simulink model "SimulinkDiagram"  (R2019a)
settings: Solver=VariableStepAuto  StartTime=0.0  StopTime=10.0  RelTol=1e-3
undefined symbols (not defined in the file): DesiredPose, DesiredTwist
libraries: simulink x4
settings Model: Creator=Amador  LastModifiedBy=Amador

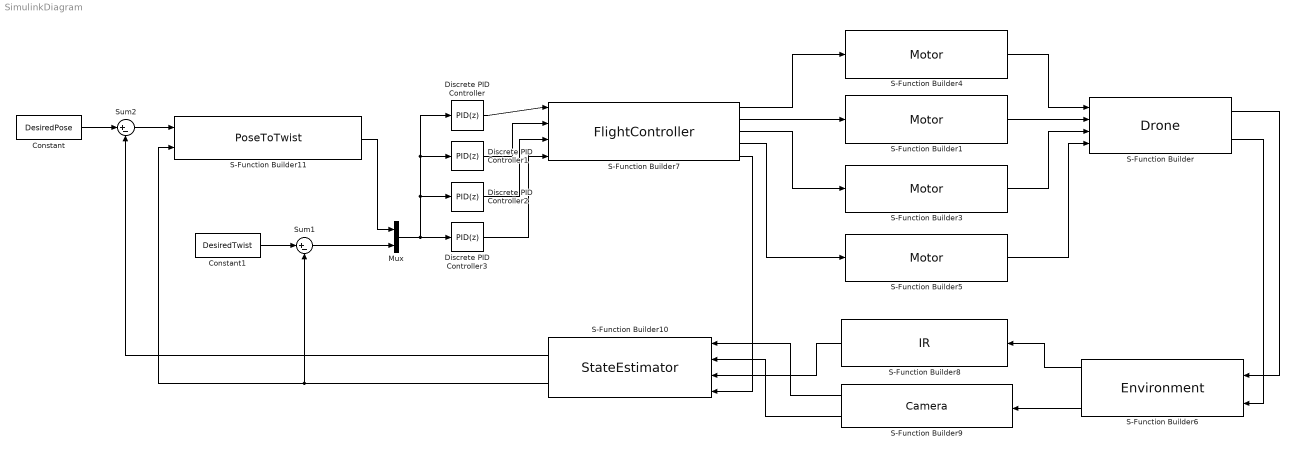
== system SimulinkDiagram ==
  Constant : Constant  Value=DesiredPose
  Constant1 : Constant  Value=DesiredTwist
  Discrete PID Controller{,1..3} (4 alike) : simulink/Continuous/PID Controller  Controller=PID  Form=Parallel  TimeDomain=Discrete-time  SampleTime=-1  IntegratorMethod=Forward Euler  FilterMethod=Forward Euler  ControllerParametersSource=internal  P=1  I=1  D=0  UseFilter=on  N=100  TunerSelectOption=Transfer Function Based (PID Tuner App)  InitialConditionSource=internal  InitialConditionForIntegrator=0  InitialConditionForFilter=0  DifferentiatorICPrevScaledInput=0  ExternalReset=none  TrackingMode=off  Kt=1  LimitOutput=off  UpperSaturationLimit=inf  LowerSaturationLimit=-inf  LinearizeAsGain=off  AntiWindupMode=none  Kb=1  POutMin=[]  POutMax=[]  IOutMin=[]  IOutMax=[]  DOutMin=[]  DOutMax=[]  NOutMin=[]  NOutMax=[]  SumOutMin=[]  SumOutMax=[]  SaturationOutMin=[]  SaturationOutMax=[]  PParamMin=[]  PParamMax=[]  IParamMin=[]  IParamMax=[]  DParamMin=[]  DParamMax=[]  NParamMin=[]  NParamMax=[]  KbParamMin=[]  KbParamMax=[]  KtParamMin=[]  KtParamMax=[]  KbOutMin=[]  KbOutMax=[]  KtOutMin=[]  KtOutMax=[]  IntegratorOutMin=[]  IntegratorOutMax=[]  FilterOutMin=[]  FilterOutMax=[]  SumI1OutMin=[]  SumI1OutMax=[]  SumI2OutMin=[]  SumI2OutMax=[]  SumI3OutMin=[]  SumI3OutMax=[]  SumI4OutMin=[]  SumI4OutMax=[]  SumDOutMin=[]  SumDOutMax=[]  DifferentiatorOutMin=[]  DifferentiatorOutMax=[]  FilterDiffOutCoefMin=[]  FilterDiffOutCoefMax=[]  ReciprocalOutMin=[]  ReciprocalOutMax=[]  SumDenOutMin=[]  SumDenOutMax=[]  SumNumOutMin=[]  SumNumOutMax=[]  DivideOutMin=[]  DivideOutMax=[]  IntegratorContinuousStateAttributes=''  IntegratorStateMustResolveToSignalObject=off  IntegratorRTWStateStorageClass=Auto  FilterContinuousStateAttributes=''  FilterStateMustResolveToSignalObject=off  FilterRTWStateStorageClass=Auto  ParallelPVariant=InternalParameters  IdealPVariant=Disabled  IVariant=InternalParameters  DVariant=InternalParameters  IntegratorVariant=Discrete  SatVariant=Disabled  AWVariant=Passthrough  PCopyVariant=Disabled  TRVariant=Disabled  FdbkBlocksVariant=Forward  IdealPFdbkVariant=Disabled  SatFdbkVariant=Disabled  DerivativeFilterVariant=ForwardEulerFilter  NVariant=InternalParameters  NCopyVariant=Disabled  FilterICVariant=InternalICsFilter  IntegratorICVariant=InternalICs  ExternalResetVariant=Disabled  TRSumVariant=Passthrough  SumFdbkVariant=Disabled  SumVariant=Sum_PID
  Mux : Mux  Inputs=2
  S-Function Builder : S-Function  InitFcn=try, set_param(gcb,'FunctionName','Drone'), end  FunctionName=Drone  SFunctionDeploymentMode=off  EnableBusSupport=off  mask(S-Function Builder){}
      mask help: Simulink:masks:SFunctionBuilder_MD
      mask init:
      | val = [[.9  0.75 0.75 1 1 .9 .9 1]',[1 1 0.75 0.75 .9 .9 1 .9]'];try , sys = get_param(gcb,'SfunBuilderFcnName');if isempty(sys), sys = get_param(gcb,'FunctionName'); end,catch, sys = get_param(gcb,'FunctionName'); end
      settings: CopyFcn=set_param(gcbh,'LinkStatus','none')  PreSaveFcn=try, set_param(gcb,'FunctionName','Drone'), end  OpenFcn=sfunctionwizard(gcbh)
      mask Display: plot(val(:,1),val(:,2)),disp(sys), port_label('input',1,'m1'), port_label('input',2,'m2'), port_label('input',3,'m3'), port_label('input',4,'m4'), port_label('output',1,'Expected Pose'), port_label('output',2,'Expected Twist')
  S-Function Builder1 : S-Function  InitFcn=try, set_param(gcb,'FunctionName','Motor'), end  FunctionName=Motor  SFunctionDeploymentMode=off  EnableBusSupport=off  mask(S-Function Builder){}
      mask help: Simulink:masks:SFunctionBuilder_MD
      mask init: same as SimulinkDiagram/S-Function Builder
      settings: CopyFcn=set_param(gcbh,'LinkStatus','none')  OpenFcn=sfunctionwizard(gcbh)
      mask Display: plot(val(:,1),val(:,2)),disp(sys), port_label('input',1,'Voltage Pulses'), port_label('output',1,'Throttle (RPM)')
  S-Function Builder10 : S-Function  InitFcn=try, set_param(gcb,'FunctionName','StateEstimator'), end  FunctionName=StateEstimator  SFunctionDeploymentMode=off  EnableBusSupport=off  mask(S-Function Builder){}
      mask help: Simulink:masks:SFunctionBuilder_MD
      mask init: same as SimulinkDiagram/S-Function Builder
      settings: CopyFcn=set_param(gcbh,'LinkStatus','none')  PreSaveFcn=try, set_param(gcb,'FunctionName','StateEstimator'), end  OpenFcn=sfunctionwizard(gcbh)
      mask Display: plot(val(:,1),val(:,2)),disp(sys), port_label('input',1,'Camera Pose'), port_label('input',2,'Camera Twist'), port_label('input',3,'Distance to Floor'), port_label('input',4,'IMU'), port_label('output',1,'Estimated Pose'), port_label('output',2,'Estimated Twist')
  S-Function Builder11 : S-Function  InitFcn=try, set_param(gcb,'FunctionName','PoseToTwist'), end  FunctionName=PoseToTwist  SFunctionDeploymentMode=off  EnableBusSupport=off  mask(S-Function Builder){}
      mask help: Simulink:masks:SFunctionBuilder_MD
      mask init: same as SimulinkDiagram/S-Function Builder
      settings: CopyFcn=set_param(gcbh,'LinkStatus','none')  PreSaveFcn=try, set_param(gcb,'FunctionName','PoseToTwist'), end  OpenFcn=sfunctionwizard(gcbh)
      mask Display: plot(val(:,1),val(:,2)),disp(sys), port_label('input',1,'Pose Difference'), port_label('input',2,'Current Twist'), port_label('output',1,'Twist Difference')
  S-Function Builder3 : S-Function  InitFcn=try, set_param(gcb,'FunctionName','Motor'), end  FunctionName=Motor  SFunctionDeploymentMode=off  EnableBusSupport=off  mask(S-Function Builder){}
      mask help: Simulink:masks:SFunctionBuilder_MD
      mask init: same as SimulinkDiagram/S-Function Builder
      settings: CopyFcn=set_param(gcbh,'LinkStatus','none')  OpenFcn=sfunctionwizard(gcbh)
      mask Display: plot(val(:,1),val(:,2)),disp(sys), port_label('input',1,'Voltage Pulses'), port_label('output',1,'Throttle (RPM)')
  S-Function Builder4 : S-Function  InitFcn=try, set_param(gcb,'FunctionName','Motor'), end  FunctionName=Motor  SFunctionDeploymentMode=off  EnableBusSupport=off  mask(S-Function Builder){}
      mask help: Simulink:masks:SFunctionBuilder_MD
      mask init: same as SimulinkDiagram/S-Function Builder
      settings: CopyFcn=set_param(gcbh,'LinkStatus','none')  OpenFcn=sfunctionwizard(gcbh)
      mask Display: plot(val(:,1),val(:,2)),disp(sys), port_label('input',1,'Voltage Pulses'), port_label('output',1,'Throttle (RPM)')
  S-Function Builder5 : S-Function  InitFcn=try, set_param(gcb,'FunctionName','Motor'), end  FunctionName=Motor  SFunctionDeploymentMode=off  EnableBusSupport=off  mask(S-Function Builder){}
      mask help: Simulink:masks:SFunctionBuilder_MD
      mask init: same as SimulinkDiagram/S-Function Builder
      settings: CopyFcn=set_param(gcbh,'LinkStatus','none')  OpenFcn=sfunctionwizard(gcbh)
      mask Display: plot(val(:,1),val(:,2)),disp(sys), port_label('input',1,'Voltage Pulses'), port_label('output',1,'Throttle (RPM)')
  S-Function Builder6 : S-Function  InitFcn=try, set_param(gcb,'FunctionName','Environment'), end  FunctionName=Environment  SFunctionDeploymentMode=off  EnableBusSupport=off  mask(S-Function Builder){}
      mask help: Simulink:masks:SFunctionBuilder_MD
      mask init: same as SimulinkDiagram/S-Function Builder
      settings: CopyFcn=set_param(gcbh,'LinkStatus','none')  PreSaveFcn=try, set_param(gcb,'FunctionName','Environment'), end  OpenFcn=sfunctionwizard(gcbh)
      mask Display: plot(val(:,1),val(:,2)),disp(sys), port_label('input',1,'Expected Pose'), port_label('input',2,'Expected Twist'), port_label('output',1,'Real Pose'), port_label('output',2,'Real Twist'), port_label('output',3,'Image')
  S-Function Builder7 : S-Function  InitFcn=try, set_param(gcb,'FunctionName','FlightController'), end  FunctionName=FlightController  SFunctionDeploymentMode=off  EnableBusSupport=off  mask(S-Function Builder){}
      mask help: Simulink:masks:SFunctionBuilder_MD
      mask init: same as SimulinkDiagram/S-Function Builder
      settings: CopyFcn=set_param(gcbh,'LinkStatus','none')  PreSaveFcn=try, set_param(gcb,'FunctionName','FlightController'), end  OpenFcn=sfunctionwizard(gcbh)
      mask Display: plot(val(:,1),val(:,2)),disp(sys), port_label('input',1,'Roll Velocity'), port_label('input',2,'Pitch Velocity'), port_label('input',3,'Yaw Velocity'), port_label('input',4,'Throttle'), port_label('output',1,'Control m1'), port_label('output',2,'Control m2'), port_label('output',3,'Control m3'), port_label('output',4,'Control m4'), port_label('output',5,'IMU Data')
  S-Function Builder8 : S-Function  InitFcn=try, set_param(gcb,'FunctionName','IR'), end  FunctionName=IR  SFunctionDeploymentMode=off  EnableBusSupport=off  mask(S-Function Builder){}
      mask help: Simulink:masks:SFunctionBuilder_MD
      mask init: same as SimulinkDiagram/S-Function Builder
      settings: CopyFcn=set_param(gcbh,'LinkStatus','none')  OpenFcn=sfunctionwizard(gcbh)
      mask Display: plot(val(:,1),val(:,2)),disp(sys), port_label('input',1,'Distance'), port_label('output',1,'Estimated Distance')
  S-Function Builder9 : S-Function  InitFcn=try, set_param(gcb,'FunctionName','Camera'), end  FunctionName=Camera  SFunctionDeploymentMode=off  EnableBusSupport=off  mask(S-Function Builder){}
      mask help: Simulink:masks:SFunctionBuilder_MD
      mask init: same as SimulinkDiagram/S-Function Builder
      settings: CopyFcn=set_param(gcbh,'LinkStatus','none')  PreSaveFcn=try, set_param(gcb,'FunctionName','Camera'), end  OpenFcn=sfunctionwizard(gcbh)
      mask Display: plot(val(:,1),val(:,2)),disp(sys), port_label('input',1,'Image'), port_label('output',1,'Estimated Pose'), port_label('output',2,'Estimated Twist')
  Sum1 : Sum  Inputs=|+-
  Sum2 : Sum  Inputs=|+-
  wires:
  S-Function Builder4/1 -> S-Function Builder/1
  S-Function Builder1/1 -> S-Function Builder/2
  S-Function Builder3/1 -> S-Function Builder/3
  S-Function Builder5/1 -> S-Function Builder/4
  S-Function Builder/1 -> S-Function Builder6/1
  S-Function Builder/2 -> S-Function Builder6/2
  S-Function Builder7/1 -> S-Function Builder4/1
  S-Function Builder7/2 -> S-Function Builder1/1
  S-Function Builder6/1 -> S-Function Builder8/1
  S-Function Builder6/3 -> S-Function Builder9/1
  S-Function Builder7/3 -> S-Function Builder3/1
  S-Function Builder7/4 -> S-Function Builder5/1
  S-Function Builder9/1 -> S-Function Builder10/1
  S-Function Builder9/2 -> S-Function Builder10/2
  S-Function Builder8/1 -> S-Function Builder10/3
  S-Function Builder7/5 -> S-Function Builder10/4
  Discrete PID Controller/1 -> S-Function Builder7/1
  Discrete PID Controller1/1 -> S-Function Builder7/2
  Discrete PID Controller2/1 -> S-Function Builder7/3
  Discrete PID Controller3/1 -> S-Function Builder7/4
  Constant1/1 -> Sum1/1
  Mux/1 -> Discrete PID Controller/1, Discrete PID Controller1/1, Discrete PID Controller2/1, Discrete PID Controller3/1
  Constant/1 -> Sum2/1
  S-Function Builder10/1 -> Sum2/2
  Sum2/1 -> S-Function Builder11/1
  S-Function Builder10/2 -> S-Function Builder11/2, Sum1/2
  S-Function Builder11/1 -> Mux/1
  Sum1/1 -> Mux/2
